simulink model "Setpoint_Controller_testslx"  (R2025a)
settings: Solver=VariableStepAuto  StartTime=0.0  StopTime=0.5  RelTol=1e-3
settings Model: Creator=Eduardoht  LastModifiedBy=Eduardoht

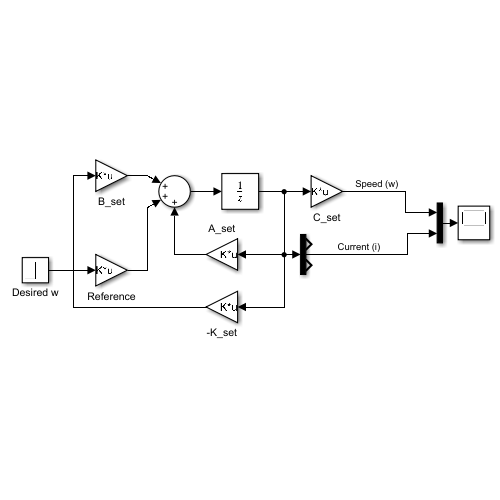
[thumbnail: Simulink's stored preview of the top-level diagram]
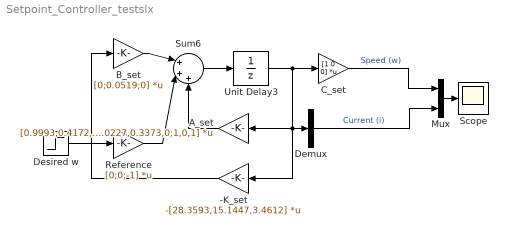
== system Setpoint_Controller_testslx ==
  -K_set : Gain  Gain=-[28.3593,15.1447,3.4612]  Multiplication=Matrix(K*u)
  A_set : Gain  Gain=[0.9993,0.4172,0;-0.0227,0.3373,0;1,0,1]  Multiplication=Matrix(K*u)
  B_set : Gain  Gain=[0;0.0519;0]  Multiplication=Matrix(K*u)
  C_set : Gain  Gain=[1 0 0]  Multiplication=Matrix(K*u)
  Demux : Demux  Outputs=3
  Desired w : Step  Time=0  After=70  SampleTime=0
  Mux : Mux  Inputs=2
  Reference : Gain  Gain=[0;0;-1]  Multiplication=Matrix(K*u)
  Scope : Scope
      settings: ActiveDisplayYMinimum=-8.7499999999999947  ActiveDisplayYMaximum=78.749999999999972
  Sum6 : Sum  Inputs=|+++
  Unit Delay3 : UnitDelay  SampleTime=0.001  HasFrameUpgradeWarning=on
  wires:
  -K_set/1 -> B_set/1
  B_set/1 -> Sum6/1
  Sum6/1 -> Unit Delay3/1
  Unit Delay3/1 -> Demux/1, -K_set/1, A_set/1, C_set/1
  C_set/1 -> Mux/1  "Speed (w)"
  Desired w/1 -> Reference/1
  A_set/1 -> Sum6/3
  Reference/1 -> Sum6/2
  Demux/2 -> Mux/2  "Current (i)"
  Mux/1 -> Scope/1
